simulink model "control"  (R2018a)
settings: Solver=VariableStepAuto  StartTime=0.0  StopTime=63  FixedStep=0.0001  RelTol=1e-3
settings Model: Creator=charlie772  LastModifiedBy=charlie772

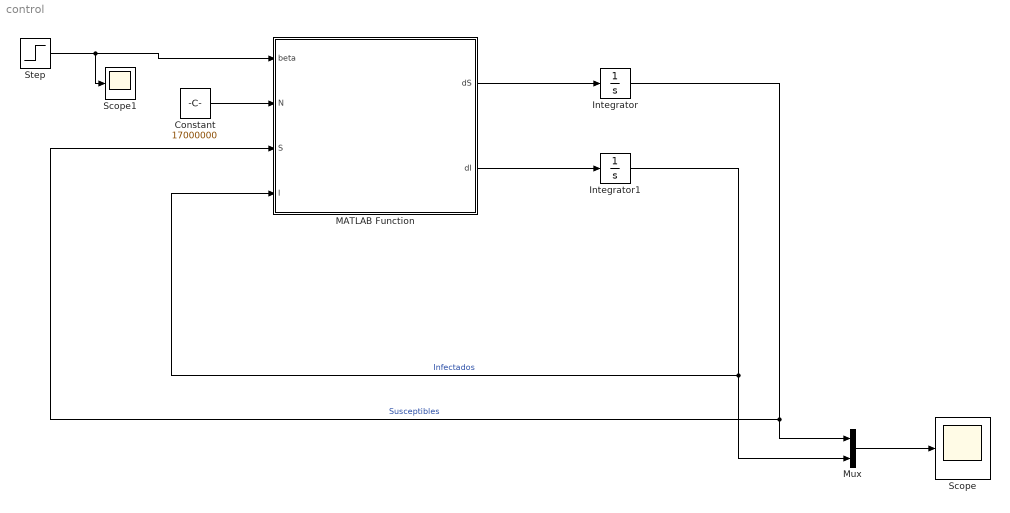
== system control ==
  Constant : Constant  Value=17000000
  Integrator : Integrator  InitialCondition=17000000
  Integrator1 : Integrator  InitialCondition=1
  MATLAB Function : MATLAB Function  TreatAsAtomicUnit=on
  Mux : Mux  Inputs=2
  Scope : Scope
  Scope1 : Scope
  Step : Step  Time=0  After=0.1399116  SampleTime=0.000001
  wires:
  MATLAB Function/1(dS) -> Integrator/1
  Integrator/1 -> Mux/1, MATLAB Function/3(S)  "Susceptibles"
  MATLAB Function/2(dI) -> Integrator1/1
  Integrator1/1 -> Mux/2, MATLAB Function/4(I)  "Infectados"
  Constant/1 -> MATLAB Function/2(N)
  Mux/1 -> Scope/1
  Step/1 -> Scope1/1, MATLAB Function/1(beta)

== matlab function control/MATLAB Function ==
  data: beta input; N input; S input; dS output; I input; dI output
function [dS,dI] = SIRD(beta,N,S,I)
gamma_r = 0.0144079;
gamma_d = 0.0047093;

dS = -(beta/N)*I* S;
dI = (beta/N)*S*I - (gamma_r+gamma_d)*I; 
end
